simulink model "TASK3_LAB"  (R2024b)
settings: Solver=ode4  StartTime=0.0  StopTime=T_SIM  FixedStep=T_s  RelTol=1e-3
values from neighbouring files (symbols this model uses):
  control_par = control_par1    [TASK1_LAB_Script.m]    (also in TASK2_LAB_SCRIPT.m = control_par4; TASK2_Scirpt.m = update_control_par(controller_index))
  controller_index = 2    [TASK2_LAB_SCRIPT.m]    (also in TASK2_Scirpt.m = 3)
  d = d_actual    (= 0.1604)    [TASK1_LAB_Script.m]    (also in TASK2_LAB_SCRIPT.m; TASK2_Scirpt.m)
  D = diag([0.8e-3, 0.8e-3, 5e-3, 0.0175/6, 0.0175/6, 0.0175/6*T_s, 0.0175/6*T_s].^2)    [TASK1_LAB_Script.m]    (also in TASK2_LAB_SCRIPT.m; TASK2_Scirpt.m)
  d_actual = 0.16040    (= 0.1604)    [TASK1_LAB_Script.m]    (also in TASK2_LAB_SCRIPT.m; TASK2_Scirpt.m)
  H_enc = [0, 0, 0, 1, 0, 0, 0 ... (first row only)    [TASK1_LAB_Script.m]    (also in TASK2_LAB_SCRIPT.m; TASK2_Scirpt.m)
  H_gyro = [0, 0, 0, 0, 0, -r_actual/d_actual, r_actual/d_actual]    [TASK1_LAB_Script.m]    (also in TASK2_LAB_SCRIPT.m; TASK2_Scirpt.m)
  H_motion_cap = [1, 0, 0, 0, 0, 0, 0 ... (first row only)    [TASK1_LAB_Script.m]    (also in TASK2_LAB_SCRIPT.m; TASK2_Scirpt.m)
  omega_M = 8    [TASK1_LAB_Script.m]    (also in TASK2_LAB_SCRIPT.m = 10; TASK2_Scirpt.m = 10)
  P_INIT_EKF = diag([0.1, 0.1, 0.2, 0.0175/6, 0.0175/6, 0.0175/6*T_s, 0.0175/6*T_s].^2)    [TASK1_LAB_Script.m]    (also in TASK2_LAB_SCRIPT.m; TASK2_Scirpt.m)
  PHI_INIT = [0;0]    [TASK1_LAB_Script.m]    (also in TASK2_LAB_SCRIPT.m; TASK2_Scirpt.m)
  Q_INIT = [-2.2; 0.7; -pi/2]    [TASK1_LAB_Script.m]    (also in TASK2_LAB_SCRIPT.m = [-1.6;-1.1;0]; TASK2_Scirpt.m = [-1.62033177494552;-1.09995932026211;-0.0877488080877385])
  r = r_actual    (= 0.03293)    [TASK1_LAB_Script.m]    (also in TASK2_LAB_SCRIPT.m; TASK2_Scirpt.m)
  R_3 = diag(([sigma_motion_capture, sigma_motion_capture, sigma_motion_capture,               sigma_enc, sigma_enc, sigma_imu]).^2)    [TASK1_LAB_Script.m]    (also in TASK2_LAB_SCRIPT.m; TASK2_Scirpt.m)
  r_actual = 0.03293    [TASK1_LAB_Script.m]    (also in TASK2_LAB_SCRIPT.m; TASK2_Scirpt.m)
  T_s = 0.04    [TASK1_LAB_Script.m]    (also in TASK2_LAB_SCRIPT.m; TASK2_Scirpt.m)
  Z_INIT_EKF = [Q_INIT; 0; 0; 0; 0]    [TASK1_LAB_Script.m]    (also in TASK2_LAB_SCRIPT.m; TASK2_Scirpt.m)
undefined symbols (not defined in the file or in its folder): p_loss, X, Y
libraries: robotlib x6, sharedtransform x2
(part 1 of 2)
settings Model: Creator=tomailoren  LastModifiedBy=pepeleonar
settings OptimizationCC: DefaultParameterBehavior=Inlined  EnhancedBackFolding=on  PassReuseOutputArgsAs=Individual arguments  ZeroExternalMemoryAtStartup=off  ZeroInternalMemoryAtStartup=off  MaxStackSize=64  OptimizeBlockOrder=speed  DifferentSizesBufferReuse=on  OptimizationCustomize=off  EfficientTunableParamExpr=on
settings DebuggingCC: ParameterTunabilityLossMsg=error
settings HardwareCC: ProdBitPerPointer=32  ProdBitPerSizeT=32  ProdBitPerPtrDiffT=32  ProdLargestAtomicFloat=None  ProdIntDivRoundTo=Undefined  ProdEndianess=Unspecified  ProdWordSize=32  ProdHWDeviceType=Generic->Unspecified (assume 32-bit Generic)
settings SFSimCC: MATLABDynamicMemAlloc=off
settings RTWCC: Description=Embedded Coder  SystemTargetFile=ert.tlc  HardwareBoard=Robot Operating System (ROS)  TLCOptions="-aInlineSetEventsForThisBaseRateFcn=TLC_FALSE -aSuppressMultiTaskScheduler=TLC_FALSE  -aRateBasedStepFcn=0"  TemplateMakefile=ert_default_tmf  Toolchain=Catkin  TargetLang=C++
settings CodeAppCC: ForceParamTrailComments=on  IgnoreCustomStorageClasses=off  OperatorAnnotations=on  SimulinkDataObjDesc=on  SFDataObjDesc=on  InsertBlockDesc=on

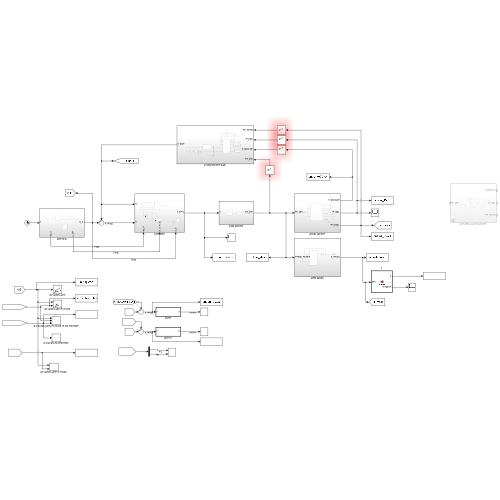
[thumbnail: Simulink's stored preview of the top-level diagram]
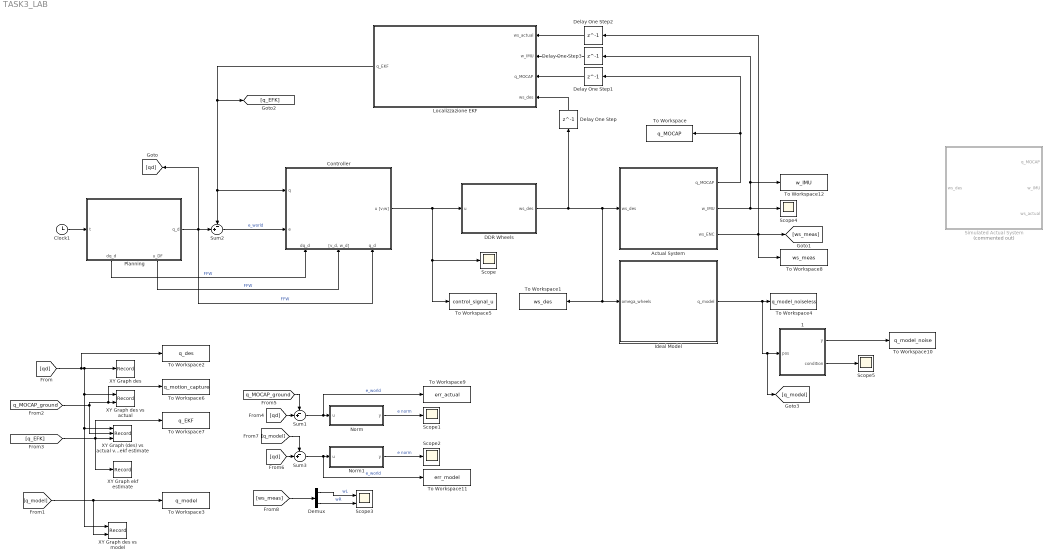
== system TASK3_LAB ==
  " 1" : MATLAB Function  TreatAsAtomicUnit=on
  Actual System : Subsystem
  Clock1 : Clock
  Controller : Subsystem
      settings: PortSchema="{\"entries\":[{\"content\":{\"sides\":[{\"content\":{\"connectorIds\":[\"In1\",\"In2\"]},\"type\":\"ConnectorPlacement.EquallySpacedRectSide\",\"uuid\":\"e15b841c-b88f-4b51-b3b6-93833098303d\"},{\"content\":{\"connectorIds\":[\"Out1\"],\"side\":\"RIGHT\"},\"type\":\"ConnectorPlacement.EquallySpacedRectSide\",\"uuid\":\"5d2a0eca-e503-49e7-9529-d06e04ddcba1\"},{\"content\":{\"side\":\"TOP\"},\"type\":\"ConnectorPlacement.EquallySpacedRectSide\",\"uuid\":\"d399d24b-56fc-4827-96f6-df142813a6e8\"},{\"content\":{\"connectorIds\":[\"In3\",\"In4\",\"In5\"],\"side\":\"BOTTOM\"},\"type\":\"ConnectorPlacement.EquallySpacedRectSide\",\"uuid\":\"6b0331a0-a5e0-48b7-9927-77bc4b376023\"}]},\"type\":\"ConnectorPlacement.EquallySpacedConnector\",\"uuid\":\"ad08f555-b948-4ebb-9107-04777bf5b8c6\"}],\"packageUris\":[\"http://schema.mathworks.com/mf0/Connector/R2020b\"],\"version\":\"1.0\"}"
  DDR Wheels : Subsystem
  Delay One Step : Delay  DelayLength=1  InitialCondition=[0;0]  SampleTime=T_s
  Delay One Step1 : Delay  DelayLength=1  InitialCondition=Q_INIT  SampleTime=T_s
  Delay One Step2 : Delay  DelayLength=1  InitialCondition=[0;0]  SampleTime=T_s
  Delay One Step3 : Delay  DelayLength=1  InitialCondition=0  SampleTime=T_s
  Demux : Demux  Outputs=2
  Ideal Model : Subsystem
  Localizzazione EKF : Subsystem
  Norm : MATLAB Function  TreatAsAtomicUnit=on
  Norm1 : MATLAB Function  TreatAsAtomicUnit=on
  Planning : Subsystem
      settings: PortSchema="{\"entries\":[{\"content\":{\"sides\":[{\"content\":{\"connectorIds\":[\"In1\"]},\"type\":\"ConnectorPlacement.EquallySpacedRectSide\",\"uuid\":\"e71c557d-01c2-4f7a-bc7e-3b96bd2d4f21\"},{\"content\":{\"connectorIds\":[\"Out1\"],\"side\":\"RIGHT\"},\"type\":\"ConnectorPlacement.EquallySpacedRectSide\",\"uuid\":\"11c737e5-20a0-46ae-a124-365c1e0e6159\"},{\"content\":{\"side\":\"TOP\"},\"type\":\"ConnectorPlacement.EquallySpacedRectSide\",\"uuid\":\"ecada992-02f9-4a2d-8aa9-74c663b4807e\"},{\"content\":{\"connectorIds\":[\"Out2\",\"Out3\"],\"side\":\"BOTTOM\"},\"type\":\"ConnectorPlacement.EquallySpacedRectSide\",\"uuid\":\"d89426e1-f636-4cd0-9f28-b48e59a8c266\"}]},\"type\":\"ConnectorPlacement.EquallySpacedConnector\",\"uuid\":\"f30e7882-f863-465d-83f6-5ea93ff1d24d\"}],\"packageUris\":[\"http://schema.mathworks.com/mf0/Connector/R2020b\"],\"version\":\"1.0\"}"
  Scope{,1..2,4..5} (5 alike) : Scope
  Scope3 : Scope  NumInputPorts=2
  Simulated Actual System : Subsystem  Commented=on
  Sum1 : Sum  Inputs=-+|
  Sum2 : Sum  Inputs=-+|
  Sum3 : Sum  Inputs=-+|
  To Workspace : ToWorkspace  VariableName=q_MOCAP  SaveFormat=Structure With Time  SampleTime=-1
  To Workspace1 : ToWorkspace  VariableName=ws_des  SaveFormat=Structure With Time  SampleTime=-1
  To Workspace10 : ToWorkspace  VariableName=q_model_noise  SaveFormat=Structure With Time  SampleTime=-1
  To Workspace11 : ToWorkspace  VariableName=err_model  SaveFormat=Structure With Time  SampleTime=-1
  To Workspace12 : ToWorkspace  VariableName=w_IMU  SaveFormat=Structure With Time  SampleTime=-1
  To Workspace2 : ToWorkspace  VariableName=q_des  SaveFormat=Structure With Time  SampleTime=-1
  To Workspace3 : ToWorkspace  VariableName=q_model  SaveFormat=Structure With Time  SampleTime=-1
  To Workspace4 : ToWorkspace  VariableName=q_model_noiseless  SaveFormat=Structure With Time  SampleTime=-1
  To Workspace5 : ToWorkspace  VariableName=control_signal_u  SaveFormat=Structure With Time  SampleTime=-1
  To Workspace6 : ToWorkspace  VariableName=q_motion_capture  SaveFormat=Structure With Time  SampleTime=-1
  To Workspace7 : ToWorkspace  VariableName=q_EKF  SaveFormat=Structure With Time  SampleTime=-1
  To Workspace8 : ToWorkspace  VariableName=ws_meas  SaveFormat=Structure With Time  SampleTime=-1
  To Workspace9 : ToWorkspace  VariableName=err_actual  SaveFormat=Structure With Time  SampleTime=-1
  XY Graph (des) vs actual vs ekf estimate : Record  FileSettingsInternal="{\"entries\":[{\"content\":{\"excelSettings\":{\"content\":{},\"type\":\"Streamout.ExcelSettings\"}},\"type\":\"Streamout.FileSettingStorage\",\"uuid\":\"\"}],\"packageUris\":[\"http:\\/\\/schema.mathworks.com\\/mf0\\/streamout_blocks\\/R2020a\"],\"version\":\"1.0\"}"  Layout=[1 1]  SignalsInternal="{\"entries\":[{\"content\":{\"signals\":[{\"content\":{\"blockPath\":[],\"dimensions\":[3,1],\"domain\":\"\",\"hasChildren\":true,\"lineColor\":\"#edb120\",\"lineWidth\":2,\"port\":1,\"sid\":[\"\"],\"signalID\":1,\"signalName\":\"From\"},\"type\":\"RecordBlkView.Signal\",\"uuid\":\"\"},{\"content\":{\"blockPath\":[],\"channel\":[1,1],\"dimensions\":[3,1],\"domain\":\"\",\"lineColor\":\"#0072bd\",\"lineWidth\":2,\"parentID\":1,\"plots\":[ 1 ],\"port\":1,\"sid\":[\"\"],\"signalID\":2,\"signalName\":\"From\"},\"type\":\"RecordBlkView.Signal\",\"uuid\":\"\"},{\"content\":{\"blockPath\":[],\"dimensions\":[3,1],\"domain\":\"\",\"hasChildren\":true,\"lineColor\":\"#77ac30\",\"lineWidth\":2,\"port\":3,\"sid\":[\"\"],\"signalID\":3,\"signalName\":\"From3\"},\"type\":\"RecordBlkView.Signal\",\"uuid\":\"\"},{\"content\":{\"blockPath\":[],\"channel\":[1,1],\"dimensions\":[3,1],\"domain\":\"\",\"lineColor\":\"#edb120\",\"lineWidth\":2,\"parentID\":3,\"plots\":[ 1 ],\"port\":3,\"sid\":[\"\"],\"signalID\":4,\"signalName\":\"From3\"},\"type\":\"RecordBlkView.Signal\",\"uuid\":\"\"},{\"content\":{\"blockPath\":[],\"dimensions\":[3],\"domain\":\"\",\"hasChildren\":true,\"lineColor\":\"#a2142f\",\"lineWidth\":2,\"port\":2,\"sid\":[\"\"],\"signalID\":5,\"signalName\":\"From2\"},\"type\":\"RecordBlkView.Signal\",\"uuid\":\"\"},{\"content\":{\"blockPath\":[],\"channel\":[1],\"dimensions\":[3],\"domain\":\"\",\"lineColor\":\"#b746ff\",\"lineWidth\":2,\"parentID\":5,\"port\":2,\"sid\":[\"\"],\"signalID\":6,\"signalName\":\"From2\"},\"type\":\"RecordBlkView.Signal\",\"uuid\":\"\"},{\"content\":{\"blockPath\":[],\"channel\":[2,1],\"dimensions\":[3,1],\"domain\":\"\",\"lineColor\":\"#0072bd\",\"lineWidth\":2,\"parentID\":1,\"plots\":[ 1 ],\"port\":1,\"sid\":[\"\"],\"signalID\":7,\"signalName\":\"From\"},\"type\":\"RecordBlkView.Signal\",\"uuid\":\"\"},{\"content\":{\"blockPath\":[],\"channel\":[3,1],\"dimensions\":[3,1],\"domain\":\"\",\"lineColor\":\"#edb120\",\"lineWidth\":2,\"parentID\":1,\"port\":1,\"sid\":[\"\"],\"signalID\":8,\"signalName\":\"From\"},\"type\":\"RecordBlkView.Signal\",\"uuid\":\"\"},{\"content\":{\"blockPath\":[],\"channel\":[2,1],\"dimensions\":[3,1],\"domain\":\"\",\"lineColor\":\"#edb120\",\"lineWidth\":2,\"parentID\":3,\"plots\":[ 1 ],\"port\":3,\"sid\":[\"\"],\"signalID\":9,\"signalName\":\"From3\"},\"type\":\"RecordBlkView.Signal\",\"uuid\":\"\"},{\"content\":{\"blockPath\":[],\"channel\":[3,1],\"dimensions\":[3,1],\"domain\":\"\",\"lineColor\":\"#a2142f\",\"lineWidth\":2,\"parentID\":3,\"port\":3,\"sid\":[\"\"],\"signalID\":10,\"signalName\":\"From3\"},\"type\":\"RecordBlkView.Signal\",\"uuid\":\"\"},{\"content\":{\"blockPath\":[],\"channel\":[2],\"dimensions\":[3],\"domain\":\"\",\"lineColor\":\"#7e2f8e\",\"lineWidth\":2,\"parentID\":5,\"port\":2,\"sid\":[\"\"],\"signalID\":11,\"signalName\":\"From2\"},\"type\":\"RecordBlkView.Signal\",\"uuid\":\"\"},{\"content\":{\"blockPath\":[],\"channel\":[3],\"dimensions\":[3],\"domain\":\"\",\"lineColor\":\"#77ac30\",\"lineWidth\":2,\"parentID\":5,\"port\":2,\"sid\":[\"\"],\"signalID\":12,\"signalName\":\"From2\"},\"type\":\"RecordBlkView.Signal\",\"uuid\":\"\"}]},\"type\":\"RecordBlkView.InputSignals\",\"uuid\":\"\"}],\"packageUris\":[\"http:\\/\\/schema.mathworks.com\\/mf0\\/streamout_blocks\\/R2020a\"],\"version\":\"1.0\"}"  VisualizationBindings="{\"xyplotplugin\":{\"info\":[{\"series\":[{\"bindingParametersList\":[{\"parameter\":\"X-Axis\",\"signalID\":2,\"signalName\":\"From(1,1)\"},{\"parameter\":\"Y-Axis\",\"signalID\":7,\"signalName\":\"From(2,1)\"}],\"seriesID\":0},{\"bindingParametersList\":[{\"parameter\":\"X-Axis\",\"signalID\":4,\"signalName\":\"From3(1,1)\"},{\"parameter\":\"Y-Axis\",\"signalID\":9,\"signalName\":\"From3(2,1)\"}],\"seriesID\":1},{\"bindingParametersList\":[{\"parameter\":\"X-Axis\",\"signalID\":2,\"signalName\":\"From(1,1)\"}],\"seriesID\":2}],\"subplotID\":1}]}}"  CompatibilityTag=XY
  XY Graph des : Record  FileSettingsInternal="{\"entries\":[{\"content\":{\"excelSettings\":{\"content\":{},\"type\":\"Streamout.ExcelSettings\"}},\"type\":\"Streamout.FileSettingStorage\",\"uuid\":\"\"}],\"packageUris\":[\"http:\\/\\/schema.mathworks.com\\/mf0\\/streamout_blocks\\/R2020a\"],\"version\":\"1.0\"}"  Layout=[1 1]  SignalsInternal="{\"entries\":[{\"content\":{\"signals\":[{\"content\":{\"blockPath\":[],\"dimensions\":[3,1],\"domain\":\"\",\"hasChildren\":true,\"lineColor\":\"#ff13a6\",\"lineWidth\":2,\"port\":1,\"sid\":[\"\"],\"signalID\":1,\"signalName\":\"From\"},\"type\":\"RecordBlkView.Signal\",\"uuid\":\"\"},{\"content\":{\"blockPath\":[],\"channel\":[1,1],\"dimensions\":[3,1],\"domain\":\"\",\"lineColor\":\"#7e2f8e\",\"lineWidth\":2,\"parentID\":1,\"plots\":[ 1 ],\"port\":1,\"sid\":[\"\"],\"signalID\":2,\"signalName\":\"From\"},\"type\":\"RecordBlkView.Signal\",\"uuid\":\"\"},{\"content\":{\"blockPath\":[],\"channel\":[2,1],\"dimensions\":[3,1],\"domain\":\"\",\"lineColor\":\"#edb120\",\"lineWidth\":2,\"parentID\":1,\"plots\":[ 1 ],\"port\":1,\"sid\":[\"\"],\"signalID\":3,\"signalName\":\"From\"},\"type\":\"RecordBlkView.Signal\",\"uuid\":\"\"},{\"content\":{\"blockPath\":[],\"channel\":[3,1],\"dimensions\":[3,1],\"domain\":\"\",\"lineColor\":\"#7e2f8e\",\"lineWidth\":2,\"parentID\":1,\"port\":1,\"sid\":[\"\"],\"signalID\":4,\"signalName\":\"From\"},\"type\":\"RecordBlkView.Signal\",\"uuid\":\"\"}]},\"type\":\"RecordBlkView.InputSignals\",\"uuid\":\"\"}],\"packageUris\":[\"http:\\/\\/schema.mathworks.com\\/mf0\\/streamout_blocks\\/R2020a\"],\"version\":\"1.0\"}"  VisualizationBindings="{\"xyplotplugin\":{\"info\":[{\"series\":[{\"bindingParametersList\":[{\"parameter\":\"X-Axis\",\"signalID\":2,\"signalName\":\"From(1,1)\"},{\"parameter\":\"Y-Axis\",\"signalID\":3,\"signalName\":\"From(2,1)\"}],\"seriesID\":0}],\"subplotID\":1}]}}"  CompatibilityTag=XY
  XY Graph des vs actual : Record  FileSettingsInternal="{\"entries\":[{\"content\":{\"excelSettings\":{\"content\":{},\"type\":\"Streamout.ExcelSettings\"}},\"type\":\"Streamout.FileSettingStorage\",\"uuid\":\"\"}],\"packageUris\":[\"http:\\/\\/schema.mathworks.com\\/mf0\\/streamout_blocks\\/R2020a\"],\"version\":\"1.0\"}"  Layout=[1 1]  SignalsInternal="{\"entries\":[{\"content\":{\"signals\":[{\"content\":{\"blockPath\":[],\"dimensions\":[3,1],\"domain\":\"\",\"hasChildren\":true,\"lineColor\":\"#ff6929\",\"lineWidth\":2,\"port\":1,\"sid\":[\"\"],\"signalID\":1,\"signalName\":\"From\"},\"type\":\"RecordBlkView.Signal\",\"uuid\":\"\"},{\"content\":{\"blockPath\":[],\"channel\":[1,1],\"dimensions\":[3,1],\"domain\":\"\",\"lineColor\":\"#d95319\",\"lineWidth\":2,\"parentID\":1,\"port\":1,\"sid\":[\"\"],\"signalID\":2,\"signalName\":\"From\"},\"type\":\"RecordBlkView.Signal\",\"uuid\":\"\"},{\"content\":{\"blockPath\":[],\"dimensions\":[3],\"domain\":\"\",\"hasChildren\":true,\"lineColor\":\"#64d413\",\"lineWidth\":2,\"port\":2,\"sid\":[\"\"],\"signalID\":3,\"signalName\":\"From2\"},\"type\":\"RecordBlkView.Signal\",\"uuid\":\"\"},{\"content\":{\"blockPath\":[],\"channel\":[1],\"dimensions\":[3],\"domain\":\"\",\"lineColor\":\"#7e2f8e\",\"lineWidth\":2,\"parentID\":3,\"port\":2,\"sid\":[\"\"],\"signalID\":4,\"signalName\":\"From2\"},\"type\":\"RecordBlkView.Signal\",\"uuid\":\"\"},{\"content\":{\"blockPath\":[],\"channel\":[2,1],\"dimensions\":[3,1],\"domain\":\"\",\"lineColor\":\"#77ac30\",\"lineWidth\":2,\"parentID\":1,\"port\":1,\"sid\":[\"\"],\"signalID\":5,\"signalName\":\"From\"},\"type\":\"RecordBlkView.Signal\",\"uuid\":\"\"},{\"content\":{\"blockPath\":[],\"channel\":[3,1],\"dimensions\":[3,1],\"domain\":\"\",\"lineColor\":\"#4dbeee\",\"lineWidth\":2,\"parentID\":1,\"port\":1,\"sid\":[\"\"],\"signalID\":6,\"signalName\":\"From\"},\"type\":\"RecordBlkView.Signal\",\"uuid\":\"\"},{\"content\":{\"blockPath\":[],\"channel\":[2],\"dimensions\":[3],\"domain\":\"\",\"lineColor\":\"#a2142f\",\"lineWidth\":2,\"parentID\":3,\"port\":2,\"sid\":[\"\"],\"signalID\":7,\"signalName\":\"From2\"},\"type\":\"RecordBlkView.Signal\",\"uuid\":\"\"},{\"content\":{\"blockPath\":[],\"channel\":[3],\"dimensions\":[3],\"domain\":\"\",\"lineColor\":\"#139fff\",\"lineWidth\":2,\"parentID\":3,\"port\":2,\"sid\":[\"\"],\"signalID\":8,\"signalName\":\"From2\"},\"type\":\"RecordBlkView.Signal\",\"uuid\":\"\"}]},\"type\":\"RecordBlkView.InputSignals\",\"uuid\":\"\"}],\"packageUris\":[\"http:\\/\\/schema.mathworks.com\\/mf0\\/streamout_blocks\\/R2020a\"],\"version\":\"1.0\"}"  VisualizationBindings="{\"xyplotplugin\":{\"info\":[{\"series\":[],\"subplotID\":1}]}}"  CompatibilityTag=XY
  XY Graph des vs model : Record  FileSettingsInternal="{\"entries\":[{\"content\":{\"excelSettings\":{\"content\":{},\"type\":\"Streamout.ExcelSettings\"}},\"type\":\"Streamout.FileSettingStorage\",\"uuid\":\"\"}],\"packageUris\":[\"http:\\/\\/schema.mathworks.com\\/mf0\\/streamout_blocks\\/R2020a\"],\"version\":\"1.0\"}"  Layout=[1 1]  SignalsInternal="{\"entries\":[{\"content\":{\"signals\":[{\"content\":{\"blockPath\":[],\"dimensions\":[3,1],\"domain\":\"\",\"hasChildren\":true,\"lineColor\":\"#fe330a\",\"lineWidth\":2,\"port\":1,\"sid\":[\"\"],\"signalID\":1,\"signalName\":\"From\"},\"type\":\"RecordBlkView.Signal\",\"uuid\":\"\"},{\"content\":{\"blockPath\":[],\"channel\":[1,1],\"dimensions\":[3,1],\"domain\":\"\",\"lineColor\":\"#0072bd\",\"lineWidth\":2,\"parentID\":1,\"port\":1,\"sid\":[\"\"],\"signalID\":2,\"signalName\":\"From\"},\"type\":\"RecordBlkView.Signal\",\"uuid\":\"\"},{\"content\":{\"blockPath\":[],\"dimensions\":[3,1],\"domain\":\"\",\"hasChildren\":true,\"lineColor\":\"#0072bd\",\"lineWidth\":2,\"port\":2,\"sid\":[\"\"],\"signalID\":3,\"signalName\":\"From1\"},\"type\":\"RecordBlkView.Signal\",\"uuid\":\"\"},{\"content\":{\"blockPath\":[],\"channel\":[1,1],\"dimensions\":[3,1],\"domain\":\"\",\"lineColor\":\"#7e2f8e\",\"lineWidth\":2,\"parentID\":3,\"port\":2,\"sid\":[\"\"],\"signalID\":4,\"signalName\":\"From1\"},\"type\":\"RecordBlkView.Signal\",\"uuid\":\"\"},{\"content\":{\"blockPath\":[],\"channel\":[2,1],\"dimensions\":[3,1],\"domain\":\"\",\"lineColor\":\"#0072bd\",\"lineWidth\":2,\"parentID\":1,\"plots\":[ 1 ],\"port\":1,\"sid\":[\"\"],\"signalID\":5,\"signalName\":\"From\"},\"type\":\"RecordBlkView.Signal\",\"uuid\":\"\"},{\"content\":{\"blockPath\":[],\"channel\":[3,1],\"dimensions\":[3,1],\"domain\":\"\",\"lineColor\":\"#fe330a\",\"lineWidth\":2,\"parentID\":1,\"port\":1,\"sid\":[\"\"],\"signalID\":6,\"signalName\":\"From\"},\"type\":\"RecordBlkView.Signal\",\"uuid\":\"\"},{\"content\":{\"blockPath\":[],\"channel\":[2,1],\"dimensions\":[3,1],\"domain\":\"\",\"lineColor\":\"#ff13a6\",\"lineWidth\":2,\"parentID\":3,\"port\":2,\"sid\":[\"\"],\"signalID\":7,\"signalName\":\"From1\"},\"type\":\"RecordBlkView.Signal\",\"uuid\":\"\"},{\"content\":{\"blockPath\":[],\"channel\":[3,1],\"dimensions\":[3,1],\"domain\":\"\",\"lineColor\":\"#fe330a\",\"lineWidth\":2,\"parentID\":3,\"port\":2,\"sid\":[\"\"],\"signalID\":8,\"signalName\":\"From1\"},\"type\":\"RecordBlkView.Signal\",\"uuid\":\"\"}]},\"type\":\"RecordBlkView.InputSignals\",\"uuid\":\"\"}],\"packageUris\":[\"http:\\/\\/schema.mathworks.com\\/mf0\\/streamout_blocks\\/R2020a\"],\"version\":\"1.0\"}"  VisualizationBindings="{\"xyplotplugin\":{\"info\":[{\"series\":[{\"bindingParametersList\":[{\"parameter\":\"Y-Axis\",\"signalID\":5,\"signalName\":\"From(2,1)\"}],\"seriesID\":0}],\"subplotID\":1}]}}"  CompatibilityTag=XY
  XY Graph ekf estimate : Record  FileSettingsInternal="{\"entries\":[{\"content\":{\"excelSettings\":{\"content\":{},\"type\":\"Streamout.ExcelSettings\"}},\"type\":\"Streamout.FileSettingStorage\",\"uuid\":\"\"}],\"packageUris\":[\"http:\\/\\/schema.mathworks.com\\/mf0\\/streamout_blocks\\/R2020a\"],\"version\":\"1.0\"}"  Layout=[1 1]  SignalsInternal="{\"entries\":[{\"content\":{\"signals\":[{\"content\":{\"blockPath\":[],\"dimensions\":[3,1],\"domain\":\"\",\"hasChildren\":true,\"lineColor\":\"#22b573\",\"lineWidth\":2,\"port\":1,\"sid\":[\"\"],\"signalID\":1,\"signalName\":\"From3\"},\"type\":\"RecordBlkView.Signal\",\"uuid\":\"\"},{\"content\":{\"blockPath\":[],\"channel\":[1,1],\"dimensions\":[3,1],\"domain\":\"\",\"lineColor\":\"#a2142f\",\"lineWidth\":2,\"parentID\":1,\"port\":1,\"sid\":[\"\"],\"signalID\":2,\"signalName\":\"From3\"},\"type\":\"RecordBlkView.Signal\",\"uuid\":\"\"},{\"content\":{\"blockPath\":[],\"channel\":[2,1],\"dimensions\":[3,1],\"domain\":\"\",\"lineColor\":\"#22b573\",\"lineWidth\":2,\"parentID\":1,\"port\":1,\"sid\":[\"\"],\"signalID\":3,\"signalName\":\"From3\"},\"type\":\"RecordBlkView.Signal\",\"uuid\":\"\"},{\"content\":{\"blockPath\":[],\"channel\":[3,1],\"dimensions\":[3,1],\"domain\":\"\",\"lineColor\":\"#0072bd\",\"lineWidth\":2,\"parentID\":1,\"port\":1,\"sid\":[\"\"],\"signalID\":4,\"signalName\":\"From3\"},\"type\":\"RecordBlkView.Signal\",\"uuid\":\"\"}]},\"type\":\"RecordBlkView.InputSignals\",\"uuid\":\"\"}],\"packageUris\":[\"http:\\/\\/schema.mathworks.com\\/mf0\\/streamout_blocks\\/R2020a\"],\"version\":\"1.0\"}"  VisualizationBindings="{\"xyplotplugin\":{\"info\":[{\"series\":[],\"subplotID\":1}]}}"  CompatibilityTag=XY
  wires:
  Controller/1(u [v;w]) -> DDR Wheels/1(u), Scope/1, To Workspace5/1
  Localizzazione EKF/1(q_EKF) -> Controller/1(q), Sum2/1, [q_EFK]
  Delay One Step/1 -> Localizzazione EKF/4(ws_des)
  Delay One Step1/1 -> Localizzazione EKF/3(q_MOCAP)
  Delay One Step2/1 -> Localizzazione EKF/1(ws_actual)
  Delay One Step3/1 -> Localizzazione EKF/2(w_IMU)
  DDR Wheels/1(ws_des) -> Actual System/1(ws_des), Ideal Model/1(omega_wheels), To Workspace1/1, Delay One Step/1
  Actual System/1(q_MOCAP) -> To Workspace/1, Delay One Step1/1
  Actual System/2(w_IMU) -> To Workspace12/1, Delay One Step3/1, Scope4/1
  Actual System/3(ws_ENC) -> [ws_meas], Delay One Step2/1, To Workspace8/1
  Clock1/1 -> Planning/1(t)
  Planning/3(u_DF) -> Controller/4("[v_d, w_d]")  "FFW"
  Sum2/1 -> Controller/2(e)  "e_world"
  Planning/1(q_d) -> [qd], Sum2/2, Controller/5(q_d)  "FFW"
  Planning/2(dq_d) -> Controller/3(dq_d)  "FFW"
  [qd] -> XY Graph des/1, XY Graph des vs actual/1, XY Graph des vs model/1, XY Graph (des) vs actual vs ekf estimate/1, To Workspace2/1
  [q_EFK] -> To Workspace7/1, XY Graph ekf estimate/1, XY Graph (des) vs actual vs ekf estimate/3
  [q_MOCAP_ground] -> To Workspace6/1, XY Graph des vs actual/2, XY Graph (des) vs actual vs ekf estimate/2
  [q_model] -> XY Graph des vs model/2, To Workspace3/1
  Norm/1(y) -> Scope1/1  "e norm"
  Sum1/1 -> To Workspace9/1, Norm/1(u)  "e_world"
  [qd] -> Sum1/2
  [q_MOCAP_ground] -> Sum1/1
  Sum3/1 -> To Workspace11/1, Norm1/1(u)  "e_world"
  [q_model] -> Sum3/1
  [qd] -> Sum3/2
  Norm1/1(y) -> Scope2/1  "e norm"
  [ws_meas] -> Demux/1
  Demux/1 -> Scope3/1  "wL"
  Demux/2 -> Scope3/2  "wR"
  " 1"/1(y) -> To Workspace10/1
  " 1"/2(condition) -> Scope5/1
  Ideal Model/1(q_model) -> [q_model], " 1"/1(pos), To Workspace4/1

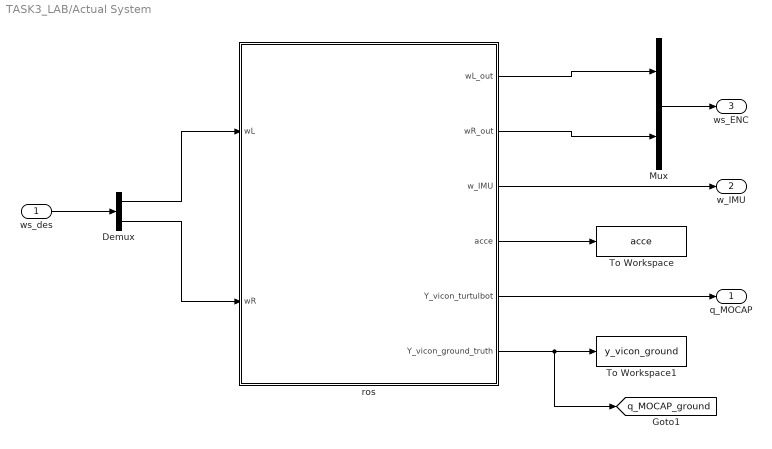
== system TASK3_LAB/Actual System ==
  ws_des : Inport
  Demux : Demux  Outputs=2
  Mux : Mux  Inputs=2
  To Workspace : ToWorkspace  VariableName=acce  SaveFormat=Structure With Time  SampleTime=-1
  To Workspace1 : ToWorkspace  VariableName=y_vicon_ground  SaveFormat=Structure With Time  SampleTime=-1
  ros : Subsystem
  q_MOCAP : Outport
  w_IMU : Outport  Port=2
  ws_ENC : Outport  Port=3
  tag scope: q_MOCAP_ground=global
  wires:
  ros/2(wR_out) -> Mux/2
  ros/4(acce) -> To Workspace/1
  ros/5(Y_vicon_turtulbot) -> q_MOCAP/1
  ros/1(wL_out) -> Mux/1
  ros/3(w_IMU) -> w_IMU/1
  ws_des/1 -> Demux/1
  Demux/1 -> ros/1(wL)
  Demux/2 -> ros/2(wR)
  Mux/1 -> ws_ENC/1
  ros/6(Y_vicon_ground_truth) -> [q_MOCAP_ground], To Workspace1/1

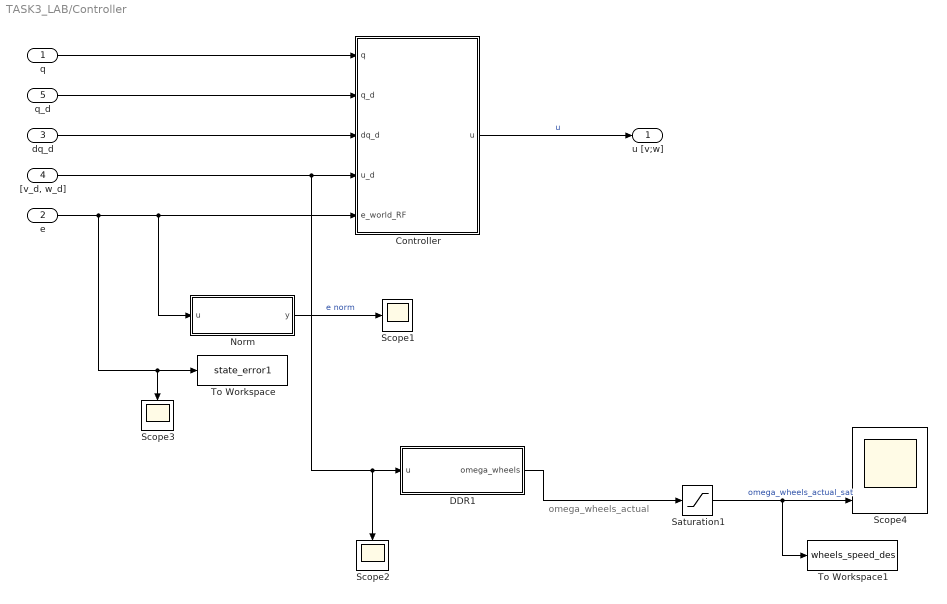
== system TASK3_LAB/Controller ==
  note: omega_wheels_actual
  q : Inport
  e : Inport  Port=2
  dq_d : Inport  Port=3
  "[v_d, w_d]" : Inport  Port=4
  q_d : Inport  Port=5
  Controller : MATLAB Function  TreatAsAtomicUnit=on
  DDR1 : MATLAB Function  TreatAsAtomicUnit=on
  Norm : MATLAB Function  TreatAsAtomicUnit=on
  Saturation1 : Saturate  UpperLimit=omega_M  LowerLimit=-omega_M
  Scope1 : Scope
  Scope2 : Scope
  Scope3 : Scope
  Scope4 : Scope  NumInputPorts=3
  To Workspace : ToWorkspace  VariableName=state_error1  SaveFormat=Structure With Time  SampleTime=-1
  To Workspace1 : ToWorkspace  VariableName=wheels_speed_des  SaveFormat=Structure With Time  SampleTime=-1
  u [v;w] : Outport
  wires:
  Saturation1/1 -> To Workspace1/1, Scope4/3  "omega_wheels_actual_sat"
  DDR1/1(omega_wheels) -> Saturation1/1
  dq_d/1 -> Controller/3(dq_d)
  Norm/1(y) -> Scope1/1  "e norm"
  e/1 -> Controller/5(e_world_RF), Norm/1(u), Scope3/1, To Workspace/1
  "[v_d, w_d]"/1 -> Controller/4(u_d), DDR1/1(u), Scope2/1
  q_d/1 -> Controller/2(q_d)
  Controller/1(u) -> u [v;w]/1  "u"
  q/1 -> Controller/1(q)

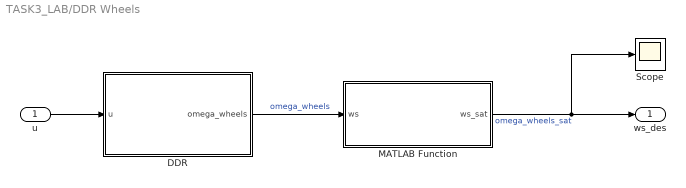
== system TASK3_LAB/DDR Wheels ==
  u : Inport
  DDR : MATLAB Function  TreatAsAtomicUnit=on
  MATLAB Function : MATLAB Function  TreatAsAtomicUnit=on
  Scope : Scope
  ws_des : Outport
  wires:
  u/1 -> DDR/1(u)
  DDR/1(omega_wheels) -> MATLAB Function/1(ws)  "omega_wheels"
  MATLAB Function/1(ws_sat) -> Scope/1, ws_des/1  "omega_wheels_sat"

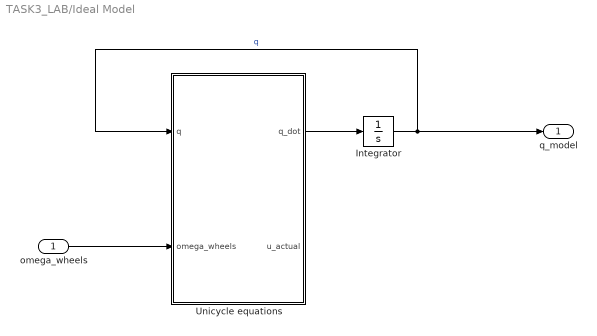
== system TASK3_LAB/Ideal Model ==
  omega_wheels : Inport
  Integrator : Integrator  InitialCondition=Q_INIT
  Unicycle equations : MATLAB Function  TreatAsAtomicUnit=on
  q_model : Outport
  wires:
  Unicycle equations/1(q_dot) -> Integrator/1
  Integrator/1 -> Unicycle equations/1(q), q_model/1  "q"
  omega_wheels/1 -> Unicycle equations/2(omega_wheels)

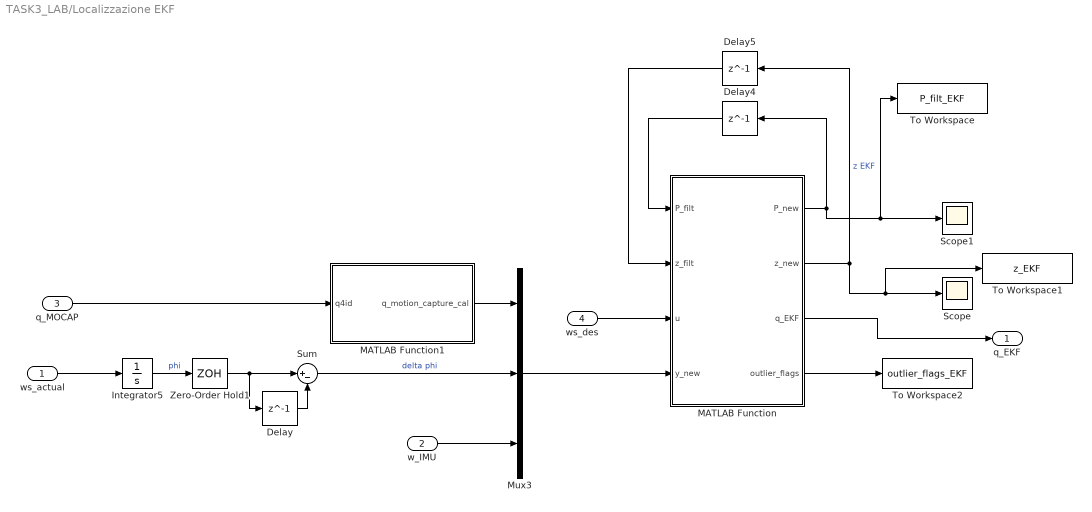
== system TASK3_LAB/Localizzazione EKF ==
  ws_actual : Inport
  w_IMU : Inport  Port=2
  q_MOCAP : Inport  Port=3
  ws_des : Inport  Port=4
  Delay : Delay  DelayLength=1  InitialCondition=[0;0]  SampleTime=T_s
  Delay4 : Delay  DelayLength=1  InitialCondition=P_INIT_EKF  SampleTime=T_s
  Delay5 : Delay  DelayLength=1  InitialCondition=Z_INIT_EKF  SampleTime=T_s
  Integrator5 : Integrator  InitialCondition=PHI_INIT
  MATLAB Function : MATLAB Function  TreatAsAtomicUnit=on
  MATLAB Function1 : MATLAB Function  TreatAsAtomicUnit=on
  Mux3 : Mux  Inputs=3
  Scope : Scope
  Scope1 : Scope
  Sum : Sum  Inputs=|+-
  To Workspace : ToWorkspace  VariableName=P_filt_EKF  SaveFormat=Structure With Time  SampleTime=-1
  To Workspace1 : ToWorkspace  VariableName=z_EKF  SaveFormat=Structure With Time  SampleTime=-1
  To Workspace2 : ToWorkspace  VariableName=outlier_flags_EKF  SaveFormat=Structure With Time  SampleTime=-1
  Zero-Order Hold1 : ZeroOrderHold  SampleTime=T_s
  q_EKF : Outport
  wires:
  ws_des/1 -> MATLAB Function/3(u)
  Mux3/1 -> MATLAB Function/4(y_new)
  MATLAB Function/3(q_EKF) -> q_EKF/1
  Delay/1 -> Sum/2
  Sum/1 -> Mux3/2  "delta phi"
  MATLAB Function/1(P_new) -> To Workspace/1, Scope1/1, Delay4/1
  MATLAB Function1/1(q_motion_capture_cal) -> Mux3/1
  MATLAB Function/2(z_new) -> To Workspace1/1, Scope/1, Delay5/1  "z EKF"
  Integrator5/1 -> Zero-Order Hold1/1  "phi"
  w_IMU/1 -> Mux3/3
  q_MOCAP/1 -> MATLAB Function1/1(q4id)
  Zero-Order Hold1/1 -> Delay/1, Sum/1
  ws_actual/1 -> Integrator5/1
  Delay5/1 -> MATLAB Function/2(z_filt)
  Delay4/1 -> MATLAB Function/1(P_filt)
  MATLAB Function/4(outlier_flags) -> To Workspace2/1

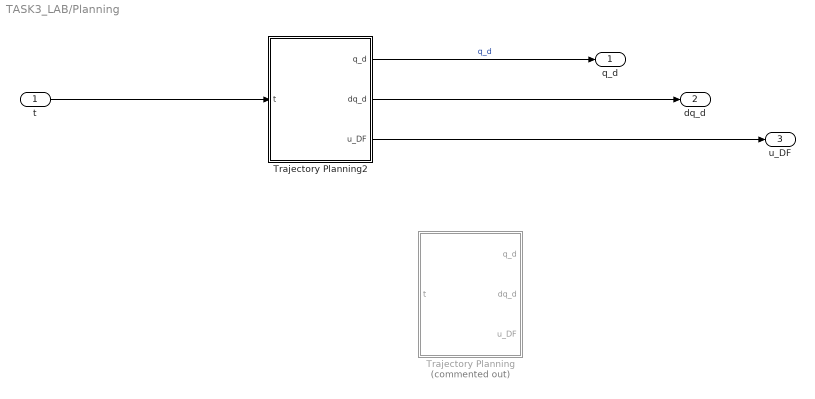
== system TASK3_LAB/Planning ==
  t : Inport
  Trajectory Planning : MATLAB Function  Commented=on  TreatAsAtomicUnit=on
  Trajectory Planning2 : MATLAB Function  TreatAsAtomicUnit=on
  q_d : Outport
  dq_d : Outport  Port=2
  u_DF : Outport  Port=3
  wires:
  Trajectory Planning2/3(u_DF) -> u_DF/1
  Trajectory Planning2/1(q_d) -> q_d/1  "q_d"
  Trajectory Planning2/2(dq_d) -> dq_d/1
  t/1 -> Trajectory Planning2/1(t)

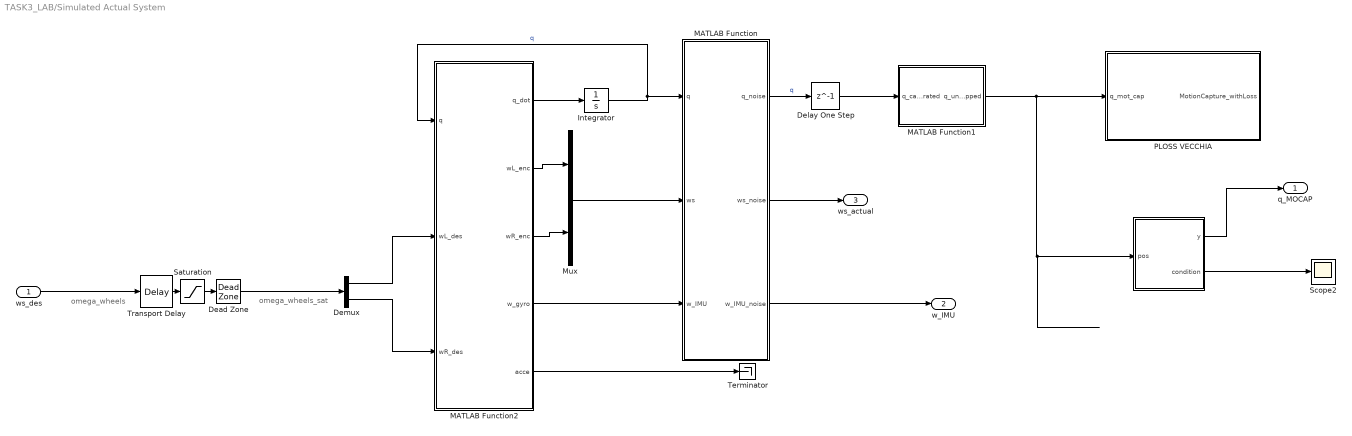
== system TASK3_LAB/Simulated Actual System ==
  note: omega_wheels_sat
  note: omega_wheels
  ws_des : Inport
  " " : MATLAB Function  TreatAsAtomicUnit=on
  Dead Zone : DeadZone  LowerValue=-0.05  UpperValue=0.05
  Delay One Step : Delay  DelayLength=1  InitialCondition=Q_INIT
  Demux : Demux  Outputs=2
  Integrator : Integrator  InitialCondition=Q_INIT
  MATLAB Function : MATLAB Function  TreatAsAtomicUnit=on
  MATLAB Function1 : MATLAB Function  TreatAsAtomicUnit=on
  MATLAB Function2 : MATLAB Function  TreatAsAtomicUnit=on
  Mux : Mux  Inputs=2
  PLOSS VECCHIA : Subsystem
  Saturation : Saturate  UpperLimit=omega_M  LowerLimit=-omega_M
  Scope2 : Scope
  Terminator : Terminator
  Transport Delay : TransportDelay  DelayTime=0.09
  q_MOCAP : Outport
  w_IMU : Outport  Port=2
  ws_actual : Outport  Port=3
  wires:
  MATLAB Function/1(q_noise) -> Delay One Step/1  "q"
  Demux/1 -> MATLAB Function2/2(wL_des)
  Demux/2 -> MATLAB Function2/3(wR_des)
  MATLAB Function2/5(acce) -> Terminator/1
  MATLAB Function2/2(wL_enc) -> Mux/1
  MATLAB Function2/3(wR_enc) -> Mux/2
  Mux/1 -> MATLAB Function/2(ws)
  MATLAB Function2/4(w_gyro) -> MATLAB Function/3(w_IMU)
  MATLAB Function/2(ws_noise) -> ws_actual/1
  MATLAB Function/3(w_IMU_noise) -> w_IMU/1
  MATLAB Function2/1(q_dot) -> Integrator/1
  Integrator/1 -> MATLAB Function2/1(q), MATLAB Function/1(q)  "q"
  " "/2(condition) -> Scope2/1
  Saturation/1 -> Dead Zone/1
  Transport Delay/1 -> Saturation/1
  ws_des/1 -> Transport Delay/1
  Dead Zone/1 -> Demux/1
  MATLAB Function1/1(q_unwrapped) -> PLOSS VECCHIA/1(q_mot_cap), " "/1(pos)
  Delay One Step/1 -> MATLAB Function1/1(q_calibrated)
  " "/1(y) -> q_MOCAP/1

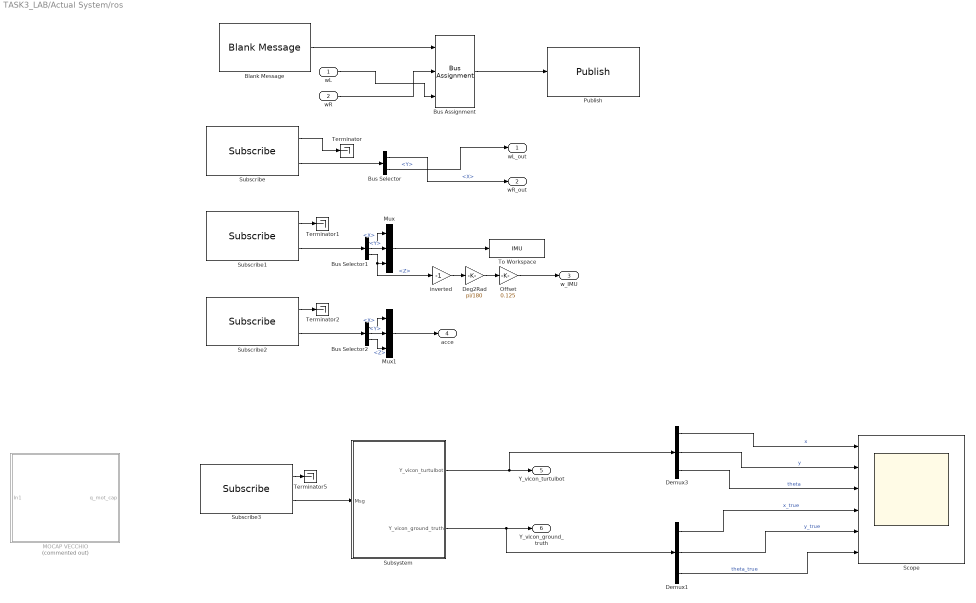
== system TASK3_LAB/Actual System/ros ==
  wL : Inport
  wR : Inport  Port=2
  Blank Message : robotlib/Blank Message  messageClass=Message  entityType=geometry_msgs/Vector3  messageType=geometry_msgs/Vector3  SampleTime=T_s  legacyBusStruct=off
  Bus Assignment : BusAssignment  AssignedSignals=X,Y
  Bus Selector : BusSelector  OutputSignals=X,Y
  Bus Selector1 : BusSelector  OutputSignals=X,Y,Z
  Bus Selector2 : BusSelector  OutputSignals=X,Y,Z
  Deg2Rad : Gain  Gain=pi/180
  Demux1 : Demux  Outputs=3
  Demux3 : Demux  Outputs=3
  MOCAP VECCHIO : Subsystem  Commented=on
  Mux : Mux  Inputs=3
  Mux1 : Mux  Inputs=3
  Offset : Gain  Gain=0.125
  Publish : robotlib/Publish  topicSource=Select from ROS network  topic=/turtlebot_01/cmd_wheels  messageType=geometry_msgs/Vector3  legacyBusStruct=off  messageQueueLength=1
  Scope : Scope  NumInputPorts=6
  Subscribe : robotlib/Subscribe  topicSource=Select from ROS network  topic=/turtlebot_01/wheelSpeeds  messageType=geometry_msgs/Vector3  SampleTime=T_s  legacyBusStruct=off  messageQueueLength=1
  Subscribe1 : robotlib/Subscribe  topicSource=Select from ROS network  topic=/turtlebot_01/gyroscope  messageType=geometry_msgs/Vector3  SampleTime=T_s  legacyBusStruct=off  messageQueueLength=1
  Subscribe2 : robotlib/Subscribe  topicSource=Select from ROS network  topic=/turtlebot_01/accelerometer  messageType=geometry_msgs/Vector3  SampleTime=T_s  legacyBusStruct=off  messageQueueLength=1
  Subscribe3 : robotlib/Subscribe  topicSource=Select from ROS network  topic=/turtlebot_01/odom  messageType=nav_msgs/Odometry  SampleTime=T_s  legacyBusStruct=off  messageQueueLength=1
  Subsystem : Subsystem
  Terminator{,1..2,5} (4 alike) : Terminator
  To Workspace : ToWorkspace  VariableName=IMU  SaveFormat=Structure With Time  SampleTime=-1
  inverted : Gain  Gain=-1
  wL_out : Outport
  wR_out : Outport  Port=2
  w_IMU : Outport  Port=3
  acce : Outport  Port=4
  Y_vicon_turtulbot : Outport  Port=5
  Y_vicon_ground_truth : Outport  Port=6
  wires:
  Subscribe2/2 -> Bus Selector2/1
  wR/1 -> Bus Assignment/2
  Bus Selector/1 -> wR_out/1  "<X>"
  Bus Selector1/2 -> Mux/2  "<Y>"
  Bus Selector2/2 -> Mux1/2  "<Y>"
  Bus Selector2/1 -> Mux1/1  "<X>"
  Bus Assignment/1 -> Publish/1
  Subscribe2/1 -> Terminator2/1
  inverted/1 -> Deg2Rad/1
  Subscribe3/1 -> Terminator5/1
  Subscribe/2 -> Bus Selector/1
  Mux1/1 -> acce/1
  Deg2Rad/1 -> Offset/1
  Bus Selector1/3 -> inverted/1, Mux/3  "<Z>"
  Offset/1 -> w_IMU/1
  wL/1 -> Bus Assignment/3
  Bus Selector1/1 -> Mux/1  "<X>"
  Bus Selector2/3 -> Mux1/3  "<Z>"
  Mux/1 -> To Workspace/1
  Subscribe/1 -> Terminator/1
  Bus Selector/2 -> wL_out/1  "<Y>"
  Subscribe1/2 -> Bus Selector1/1
  Subscribe1/1 -> Terminator1/1
  Blank Message/1 -> Bus Assignment/1
  Subscribe3/2 -> Subsystem/1(Msg)
  Demux1/2 -> Scope/5  "y_true"
  Subsystem/1(Y_vicon_turtulbot) -> Demux3/1, Y_vicon_turtulbot/1
  Subsystem/2(Y_vicon_ground_truth) -> Y_vicon_ground_truth/1, Demux1/1
  Demux3/3 -> Scope/3  "theta"
  Demux1/1 -> Scope/4  "x_true"
  Demux3/1 -> Scope/1  "x"
  Demux1/3 -> Scope/6  "theta_true"
  Demux3/2 -> Scope/2  "y"

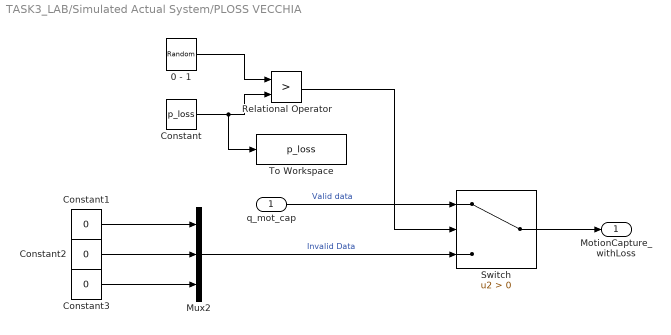
== system TASK3_LAB/Simulated Actual System/PLOSS VECCHIA ==
  q_mot_cap : Inport
  0 - 1 : UniformRandomNumber  Minimum=0  SampleTime=T_s
  Constant : Constant  Value=p_loss
  Constant1 : Constant  Value=0
  Constant2 : Constant  Value=0
  Constant3 : Constant  Value=0
  Mux2 : Mux  Inputs=3
  Relational Operator : RelationalOperator  Operator=>  OutDataTypeStr=boolean  RndMeth=Simplest  InputSameDT=off
  Switch : Switch  Criteria=u2 > Threshold  SaturateOnIntegerOverflow=off  InputSameDT=off
  To Workspace : ToWorkspace  VariableName=p_loss  SaveFormat=Structure  SampleTime=-1
      settings: Save2DSignal=2-D array (concatenate along first dimension)
  MotionCapture_withLoss : Outport
  wires:
  0 - 1/1 -> Relational Operator/1
  Constant/1 -> To Workspace/1, Relational Operator/2
  Switch/1 -> MotionCapture_withLoss/1
  Relational Operator/1 -> Switch/2
  Constant2/1 -> Mux2/2
  Mux2/1 -> Switch/3  "Invalid Data"
  Constant1/1 -> Mux2/1
  q_mot_cap/1 -> Switch/1  "Valid data"
  Constant3/1 -> Mux2/3

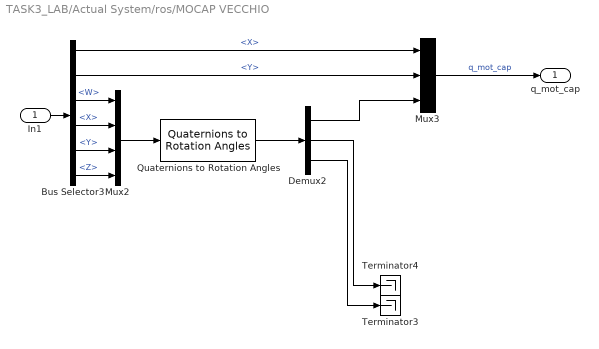
== system TASK3_LAB/Actual System/ros/MOCAP VECCHIO ==
  In1 : Inport
  Bus Selector3 : BusSelector  OutputSignals=Pose.Pose.Position.X,Pose.Pose.Position.Y,Pose.Pose.Orientation.W,Pose.Pose.Orientation.X,Pose.Pose.Orientation.Y,Pose.Pose.Orientation.Z
  Demux2 : Demux  Outputs=3
  Mux2 : Mux
  Mux3 : Mux  Inputs=3
  Quaternions to Rotation Angles : sharedtransform/Quaternions to Rotation Angles  rotationOrder=ZYX  aMode=aMode
  Terminator3 : Terminator
  Terminator4 : Terminator
  q_mot_cap : Outport
  wires:
  Bus Selector3/3 -> Mux2/1  "<W>"
  Demux2/2 -> Terminator4/1
  Quaternions to Rotation Angles/1 -> Demux2/1
  Mux3/1 -> q_mot_cap/1  "q_mot_cap"
  Bus Selector3/4 -> Mux2/2  "<X>"
  Demux2/1 -> Mux3/3
  Mux2/1 -> Quaternions to Rotation Angles/1
  Bus Selector3/1 -> Mux3/1  "<X>"
  Demux2/3 -> Terminator3/1
  Bus Selector3/2 -> Mux3/2  "<Y>"
  Bus Selector3/5 -> Mux2/3  "<Y>"
  Bus Selector3/6 -> Mux2/4  "<Z>"
  In1/1 -> Bus Selector3/1

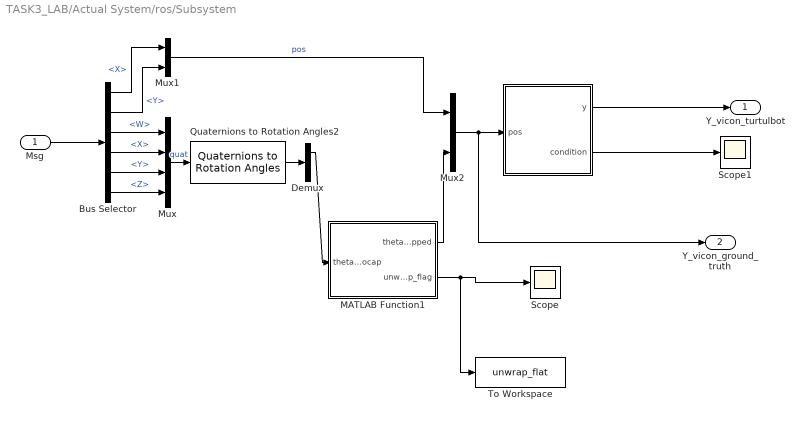
== system TASK3_LAB/Actual System/ros/Subsystem ==
  Msg : Inport
  " " : MATLAB Function  TreatAsAtomicUnit=on
  Bus Selector : BusSelector  OutputSignals=Pose.Pose.Position.X,Pose.Pose.Position.Y,Pose.Pose.Orientation.W,Pose.Pose.Orientation.X,Pose.Pose.Orientation.Y,Pose.Pose.Orientation.Z
  Demux : Demux  Outputs=3
  MATLAB Function1 : MATLAB Function  TreatAsAtomicUnit=on
  Mux : Mux
  Mux1 : Mux  Inputs=2
  Mux2 : Mux  Inputs=2
  Quaternions to Rotation Angles2 : sharedtransform/Quaternions to Rotation Angles  rotationOrder=ZYX  aMode=aMode
  Scope : Scope
  Scope1 : Scope
  To Workspace : ToWorkspace  VariableName=unwrap_flat  SaveFormat=Structure With Time  SampleTime=-1
  Y_vicon_turtulbot : Outport
  Y_vicon_ground_truth : Outport  Port=2
  wires:
  Msg/1 -> Bus Selector/1
  Mux2/1 -> Y_vicon_ground_truth/1, " "/1(pos)
  Bus Selector/3 -> Mux/1  "<W>"
  Mux/1 -> Quaternions to Rotation Angles2/1  "quat"
  Bus Selector/2 -> Mux1/2  "<Y>"
  Bus Selector/6 -> Mux/4  "<Z>"
  Bus Selector/1 -> Mux1/1  "<X>"
  " "/1(y) -> Y_vicon_turtulbot/1
  Bus Selector/4 -> Mux/2  "<X>"
  Bus Selector/5 -> Mux/3  "<Y>"
  " "/2(condition) -> Scope1/1
  MATLAB Function1/1(theta_unwrapped) -> Mux2/2
  Mux1/1 -> Mux2/1  "pos"
  Quaternions to Rotation Angles2/1 -> Demux/1
  Demux/1 -> MATLAB Function1/1(theta_mocap)
  MATLAB Function1/2(unwrap_flag) -> To Workspace/1, Scope/1

== matlab function TASK3_LAB/DDR Wheels/MATLAB Function ==
  data: ws input; ws_sat output; omega_M parameter
function ws_sat = rescaling_saturation(ws, omega_M)
    
    % to avoid a saturation of both the wheels to max value (10)
    % lost of control !


    wL = ws(1); 
    wR = ws(2);

    max_w = max(abs(wL), abs(wR));

    if max_w > omega_M
        wL_sat = wL * (omega_M / max_w);
        wR_sat = wR * (omega_M / max_w);
    else
        wL_sat = wL;
        wR_sat = wR;
    end

    ws_sat = [wL_sat; wR_sat];
end

== matlab function TASK3_LAB/Simulated Actual System/  ==
  data: y output; pos input; condition output
function [y, condition] = check(pos)

x1 = -2.9; y1 = -1.5;
x2 = -1.6; y2 = -1.1;
x3 = -1.5; y3 = -0.7;
x4 = -1.4; y4 = -0.3;
x5 = -0.6; y5 =  0.1;
x6 =  0.2; y6 =  1.5;
x7 =  1.0;
x8 =  1.1;
x9 =  2.9;

P_loss = 0.9;


if ((pos(1) >= x5) && (pos(1) <= x6)) && ((pos(2) >= y1) && (pos(2) <= y5))
    % add noise
    y = pos + 0.02*randn(3,1);
    condition = 1;
elseif ((pos(1) >= x7 ) && (pos(1) <= x9)) && ((pos(2) >= y1) && (pos(2) <= y6))
    % measurement loss
    if rand > P_loss
        y = pos;
    else
        y = 0*pos;
    end
    condition = 2;
else
    y = pos;
    condition = 0;
end

== matlab function TASK3_LAB/Norm ==
  data: u input; y output
function y = fcn(u)

y = sqrt(sum(u(1:2).^2));

== matlab function TASK3_LAB/DDR Wheels/DDR ==
  data: u input; omega_wheels output; r parameter; d parameter
function omega_wheels = kin2omegawheels(u, r, d)
omega_l = u(1)/r-d/(2*r)*u(2);
omega_r = u(1)/r+d/(2*r)*u(2);
omega_wheels = [omega_l;omega_r];

== matlab function TASK3_LAB/Norm1 ==
  data: u input; y output
function y = fcn(u)

y = sqrt(sum(u(1:2).^2));

== matlab function TASK3_LAB/Simulated Actual System/MATLAB Function1 ==
  data: q_calibrated input; q_unwrapped output
function q_unwrapped = fcn(q_calibrated)
    % Questa funzione esegue l'unwrap online della componente theta 
    % della posa calibrata del robot, rendendo il segnale continuo per il Kalman.
    
    % Pre-allochiamo l'uscita uguale all'ingresso
    q_unwrapped = q_calibrated;
    
    % Definiamo le variabili persistenti per mantenere la memoria tra i passi
    persistent theta_old N_turns first_run
    
    % Inizializzazione al primissimo passo di simulazione (t = 0)
    if isempty(first_run)
        theta_old = q_calibrated(3);
        N_turns = 0;
        first_run = false;
    end
    
    % Estraiamo il theta corrente (wrappato tra -pi e pi)
    theta_current = q_calibrated(3);
    
    % Calcoliamo la variazione rispetto al passo precedente
    delta = theta_current - theta_old;
    
    % --- ALGORITMO DI UNWRAP ONLINE ---
    % Se il robot attraversa la barriera da pi a -pi (giro in senso antiorario),
    % delta sarà circa -2*pi. Quindi intercettiamo se delta < -pi
    if delta < -pi
        N_turns = N_turns + 1;
        
    % Se il robot attraversa la barriera da -pi a pi (giro in senso orario),
    % delta sarà circa +2*pi. Quindi intercettiamo se delta > pi
    elseif delta > pi
        N_turns = N_turns - 1;
    end
    
    % Memorizziamo il valore corrente per il prossimo passo temporale
    theta_old = theta_current;
    
    % Ricostruiamo il theta continuo sommando i giri da 2*pi accumulati
    q_unwrapped(3) = theta_current + N_turns * 2 * pi;
end

== matlab function TASK3_LAB/Actual System/ros/Subsystem/MATLAB Function1 ==
  data: theta_mocap input; theta_unwrapped output; unwrap_flag output
function [theta_unwrapped, unwrap_flag] = Unwrap(theta_mocap)
    % Define persistent variables for state memory
    persistent theta_prev_mocap theta_prev_unwrapped
    
    unwrap_flag = 0;

    % Initialization at time t=0
    if isempty(theta_prev_unwrapped)
        if isnan(theta_mocap)
            theta_mocap =0;
        end
        theta_prev_mocap = theta_mocap;
        theta_prev_unwrapped = theta_mocap;
    end
    
    if isnan(theta_mocap)
        theta_unwrapped = theta_prev_unwrapped;
        unwrap_flag = 1;
        return;
    end

    delta_theta = theta_mocap - theta_prev_mocap;
    delta_wrapped = atan2(sin(delta_theta), cos(delta_theta));

    if abs(delta_wrapped)>0.5
        theta_unwrapped = theta_prev_unwrapped;
        unwrap_flag = 2;
        return;
    end
    
    theta_unwrapped = theta_prev_unwrapped + delta_wrapped;
    
    % 4. Update internal states for the next integration step
    theta_prev_unwrapped = theta_unwrapped;
    theta_prev_mocap = theta_mocap;
end

== matlab function TASK3_LAB/Planning/Trajectory Planning2 ==
  data: t input; q_d output; dq_d output; u_DF output; T_circ parameter
function [q_d, dq_d, u_DF] = get_circualt_traj_TASK3(t, T_circ)
   
    % center
    x_c = 2.0;     % x10-x9 /2
    y_c = 0.0;

    x8 = 1.45;
    y4 = -0.30;


    % Raggio e angolo iniziale (calcolati dal punto di partenza)
    r = sqrt((x8 - x_c)^2 + (y4 - y_c)^2);
    phi0 = atan2(y4 - y_c, x8 - x_c);

    % theta_start = phi0 + pi/2;   % orientation tangent to the circle in (x8,y4)
       
    % 1.5 giri = 3*pi rad in T_trj secondi
    omega = 3 * pi / T_circ;   % constant ang vel

    theta_prime = omega * t;
    phi         = phi0 + theta_prime;

    q_d  = [x_c + r*cos(phi);
            y_c + r*sin(phi);
            phi + pi/2];

    dq_d = [-omega*r*sin(phi);
             omega*r*cos(phi);
             omega];

    u_DF = [omega*r; omega];

end

== matlab function TASK3_LAB/ 1 ==
  settings: updateMethod=DISCRETE
  data: y output; pos input; condition output
function [y, condition] = check(pos)

x1 = -2.9; y1 = -1.5;
x2 = -1.6; y2 = -1.1;
x3 = -1.5; y3 = -0.7;
x4 = -1.4; y4 = -0.3;
x5 = -0.6; y5 =  0.1;
x6 =  0.2; y6 =  1.5;
x7 =  1.0;
x8 =  1.1;
x9 =  2.9;

P_loss = 0.9;


if ((pos(1) >= x5) && (pos(1) <= x6)) && ((pos(2) >= y1) && (pos(2) <= y5))
    % add noise
    y = pos + 0.02*randn(3,1);
    condition = 1;
elseif ((pos(1) >= x7 ) && (pos(1) <= x9)) && ((pos(2) >= y1) && (pos(2) <= y6))
    % measurement loss
    if rand > P_loss
        y = pos;
    else
        y = 0*pos;
    end
    condition = 2;
else
    y = pos;
    condition = 0;
end

== matlab function TASK3_LAB/Controller/Controller ==
  data: q input; q_d input; dq_d input; u_d input; u output; e_world_RF input; control_par parameter; controller_index parameter
function u = fcn(q, q_d, dq_d, u_d, e_world_RF, control_par, controller_index)

    % LINREAR controller
    if controller_index == 1
                
        vd = u_d(1); wd = u_d(2);

        % derive control matrix K
        K = linear_gains(control_par, vd, wd);
        k1 = K(1); k2 = K(2); k3 = K(3);

        % rotation of the error
        e_body = error_rotation(e_world_RF, q);
        e1 = e_body(1); e2 = e_body(2); e3 = e_body(3);

        e3 = atan2(sin(e_body(3)), cos(e_body(3)));
    
        % Linear Contrl Law
        % Define u_aux_1, u_aux_2 auxiliar inputs
        u1_aux = -k1 * e1;
        u2_aux = -k2 * e2 - k3 * e3;
        
        % 3. Real model inputs    
        v = vd * cos(e3) - u1_aux;
        w = wd - u2_aux;
        
        % Saturation (if i want a saturation directly on v and w
        % v = max(min(v, 1.5), -1.5); 
        % w = max(min(w, 3.0), -3.0);
        
        u = [v; w];


    % --------------------------------------
    % NON LINEAR controller
    elseif controller_index == 2
        
        vd = u_d(1); wd = u_d(2);

        % derive control matrix K
        K = NL_gains(control_par, vd, wd);
        k1 = K(1); k2 = K(2); k3 = K(3); 

        % rotation of the error
        e_body = error_rotation(e_world_RF, q);
        e1 = e_body(1); e2 = e_body(2); e3 = e_body(3); 
 
    
        % NON-Linear Contrl Law
        
        % Singularity: sinc(e3) = sin(e3)/e3
        if abs(e3) < 1e-1
            sinc_e3 = 1;
        else
            sinc_e3 = sin(e3)/e3;
        end
        
        % Define u_aux_1, u_aux_2 auxiliar inputs
        u1_aux = -k1 * e1;
        u2_aux = -k2 * vd * sinc_e3 * e2 - k3 * e3;
       
        % Real model inputs
        v = vd * cos(e3) - u1_aux;
        w = wd - u2_aux;
        
        % Saturation  
        % v = max(min(v, 1.5), -1.5); 
        % w = max(min(w, 3.0), -3.0);
        
        u = [v; w];


    % --------------------------------------
    % FEEDBACK LINEARIZATION (OUTPUT ERROR FB)
    elseif controller_index == 3
    % the input is q_Bd and q_Bdot

    theta = q(3);
    k1 = control_par(1); k2 = control_par(2); b = control_par(3);

    % build K matrix
    K = [k1 , 0 ; 0 , k2];

    % ep is the error of the point B
    % I just need the the first 2 components of the error (ep_x, ep_y)
    % in the world frame
    ep = [ e_world_RF(1) ; e_world_RF(2) ];

    pBd_dot = [dq_d(1); dq_d(2)];
    
    T_inv = [cos(theta),       sin(theta);
             -(1/b) * sin(theta), (1/b) * cos(theta)];

    u = T_inv * (pBd_dot + K * ep);     % u = [v; w]


    % elseif controller_index == 3
    % 
    %     theta = q(3);
    %     theta_d = q_d(3);
    %     wd = u_d(2);
    %     k1 = control_par(1); k2 = control_par(2); b = control_par(3);
    % 
    %     % build K matrix
    %     K = [k1 , 0 ; 0 , k2];
    % 
    %     % I just need the the first 2 components of the error (ep_x, ep_y)
    %     % in the world frame
    %     ep = [ e_world_RF(1) ; e_world_RF(2) ];
    % 
    %     % Translation of desired trajectory for the B-point 
    %     p_Bd = [q_d(1) + b * cos(theta_d);
    %             q_d(2) + b * sin(theta_d)];
    % 
    %     pBd_dot = [dq_d(1) - b * sin(theta_d) * wd;
    %                dq_d(2) + b * cos(theta_d) * wd];
    % 
    %     T_inv = [cos(theta),       sin(theta);
    %              -(1/b) * sin(theta), (1/b) * cos(theta)];
    % 
    %     u = T_inv * (pBd_dot + K * ep);     % u = [v; w]

    else
        u = u_d;
    end
end

% ------------------------------------------------------------------

% LOCAL FUNCTIONS


function e_body = error_rotation(e_w, q)

    % Extracts the current robot orientation
    theta = q(3);
    
    % Normalize the orientation error (3rd component) to be within [-pi, pi]
    % This prevents the robot from making unnecessary 360-degree turns.
    e_theta = e_w(3);
    e_w(3) = atan2(sin(e_theta), cos(e_theta));
    
    % Rotation matrix transpose
    R_T = [ cos(theta), sin(theta), 0;
           -sin(theta), cos(theta), 0;
                0,          0,      1];
            
    % Compute error in Body Frame
    e_body = R_T * e_w;

end
    
function K = linear_gains(control_par, vd, wd)
    xi = control_par(1);
    a = control_par(2);

    k1 = 2 * xi * a; 
    k3 = k1;
    
    % if vd is zero the gain will be huge (controlled then by saturation)
    if abs(vd) < 1e-4
        if vd >= 0
            vd = 1e-4;
        else
            vd = -1e-4;
        end
    end
        
    k2 = (a^2 - wd^2)/vd;

    K = [k1; k2; k3];
end


function K = NL_gains(control_par, vd, wd)
    xi = control_par(1);
    b = control_par(2);

    k1 = 2 * xi * sqrt(b*vd + wd^2); 
    k3 = k1;
    k2 = b;

    K = [k1; k2; k3];
end

== matlab function TASK3_LAB/Controller/DDR1 ==
  data: u input; omega_wheels output; r_actual parameter; d_actual parameter
function omega_wheels = kin2omegawheels(u, r_actual, d_actual)
omega_l = u(1)/r_actual-d_actual/(2*r_actual)*u(2);
omega_r = u(1)/r_actual+d_actual/(2*r_actual)*u(2);
omega_wheels = [omega_l;omega_r];

== matlab function TASK3_LAB/Controller/Norm ==
  data: u input; y output
function y = fcn(u)

y = sqrt(sum(u(1:2).^2));

== matlab function TASK3_LAB/Ideal Model/Unicycle equations ==
  data: q input; omega_wheels input; q_dot output; r_actual parameter; d_actual parameter; u_actual output
function [q_dot, u_actual] = q_dot(q, omega_wheels, r_actual, d_actual)
    
    u_actual = [r_actual/2, r_actual/2;-r_actual/d_actual, r_actual/d_actual]*omega_wheels;
    
    theta = q(3);

    q_dot = [[cos(theta), 0];[sin(theta), 0];[0,1]] * u_actual;

== matlab function TASK3_LAB/Simulated Actual System/MATLAB Function ==
  settings: updateMethod=DISCRETE
  data: q input; q_noise output; ws input; w_IMU input; ws_noise output; w_IMU_noise output; D parameter
function [q_noise, ws_noise, w_IMU_noise] = fcn(q, ws, w_IMU, D)

    % --- DEVIAZIONI STANDARD (sigma) ---
    
    % Deviazioni per il modello (q)
    sigma_x     = D(1,1); 
    sigma_y     = D(2,2);
    sigma_theta = D(3,3); 
    sigma_ws    = D(6,6); 
    sigma_w_IMU = 0.01;      
    % sigma_x     = 5e-3; 
    % sigma_y     = 5e-3;
    % sigma_theta = 5e-2; 
    % sigma_ws    = 1e-1; 
    % sigma_w_IMU = 2e-2;
    
    % --- GENERAZIONE RUMORE STATO (q) ---
    % Moltiplica per sigma, non per sigma^2
    x_n = q(1) + sigma_x * randn;
    y_n = q(2) + sigma_y * randn;
    
    % Prima aggiungi il rumore, POI wrappi l'angolo
    theta_noisy = q(3) + sigma_theta * randn;
    theta_n = atan2(sin(theta_noisy), cos(theta_noisy));
    
    q_noise = [x_n; y_n; theta_n];
    
    % --- GENERAZIONE RUMORE SENSORI ---
    ws_noise    = ws    + sigma_ws    * randn(size(ws));
    w_IMU_noise = w_IMU + sigma_w_IMU * randn(size(w_IMU));

end

== matlab function TASK3_LAB/Localizzazione EKF/MATLAB Function1 ==
  data: q4id input; q_motion_capture_cal output
function q_motion_capture_cal = calibration(q4id)

x_off_cal = -0.00434;
y_off_cal = -0.00361;
theta_off = 0.02331;


theta_cal = q4id(3) - theta_off;
x_cal = q4id(1) - (x_off_cal * cos(theta_cal) - y_off_cal * sin(theta_cal));
y_cal = q4id(2) - (x_off_cal * sin(theta_cal) + y_off_cal * cos(theta_cal));


q_motion_capture_cal = [x_cal; y_cal; theta_cal];

== matlab function TASK3_LAB/Simulated Actual System/MATLAB Function2 ==
  data: q input; q_dot output; wL_des input; wR_des input; wL_enc output; wR_enc output; w_gyro output; r parameter; d parameter; T_s parameter; acce output
function [q_dot, wL_enc, wR_enc, w_gyro, acce] = robot_simulator(q, wL_des, wR_des, r, d, T_s)
    
    wL_enc = wL_des;
    wR_enc = wR_des;
      
    v = (r/2) * (wR_des + wL_des);
    omega = (r/d) * (wR_des - wL_des);
    
    w_gyro = -omega;
    
    q_dot= zeros(3,1);
    
    q_dot(1) = v*cos(q(3));
    q_dot(2) = v*sin(q(3));
    q_dot(3) = omega;

    acce = [0;0;0];
    
end
